simulink model "angleControllerValidation"  (R2021b)
settings: Solver=VariableStepAuto  StartTime=0.0  StopTime=10.0  RelTol=1e-3
values from neighbouring files (symbols this model uses):
  B_x = 12    [XthetaControllers.m]    (also in x_model_sheet.m)
  J_x = 0.13    [XthetaControllers.m]    (also in x_model_sheet.m)
  r_x = 75e-3    (= 0.075)    [XthetaControllers.m]    (also in x_model_sheet.m)
undefined symbols (not defined in the file or in its folder): cFrictionX, InitWireLength, InitXPos, k_ex, m_l, m_t, sFrictionX, Xref
settings Model: Creator=bosto  LastModifiedBy=bosto

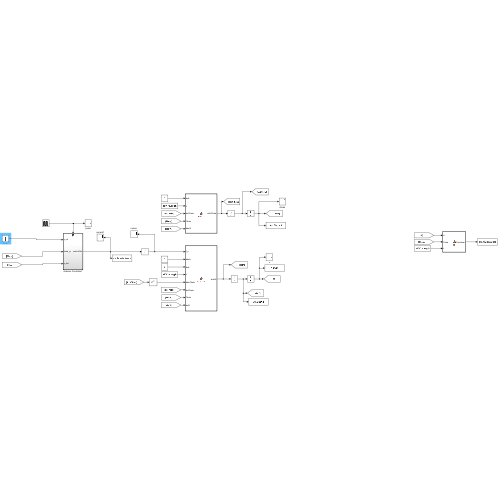
[thumbnail: Simulink's stored preview of the top-level diagram]
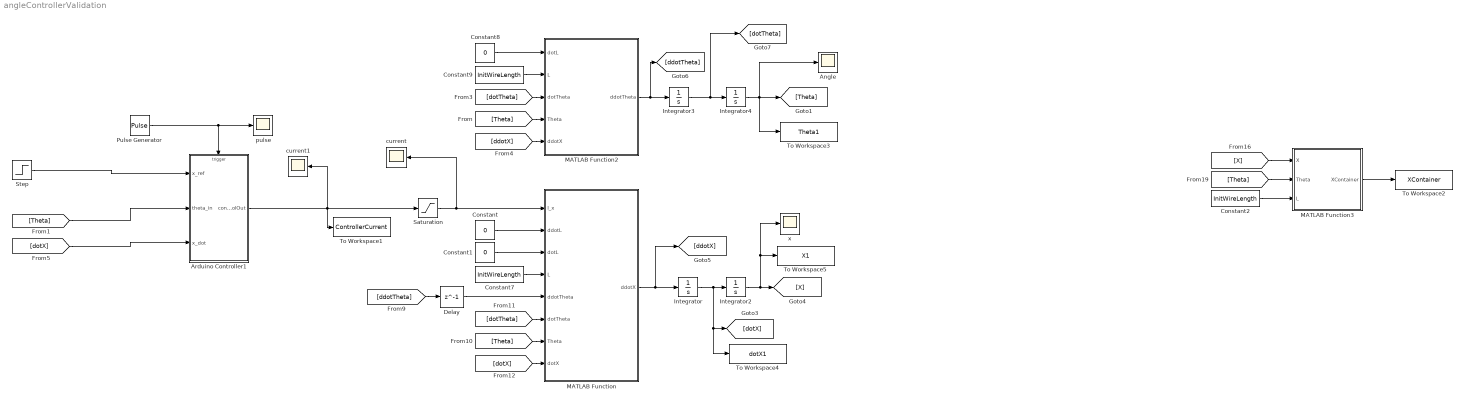
== system angleControllerValidation ==
  Angle : Scope
  Arduino Controller1 : Subsystem
  Constant : Constant  Value=0
  Constant1 : Constant  Value=0
  Constant2 : Constant  Value=InitWireLength
  Constant7 : Constant  Value=InitWireLength
  Constant8 : Constant  Value=0
  Constant9 : Constant  Value=InitWireLength
  Delay : Delay  DelayLength=1  InitialCondition=0
  Integrator : Integrator
  Integrator2 : Integrator  InitialCondition=InitXPos
  Integrator3 : Integrator
  Integrator4 : Integrator
  MATLAB Function : MATLAB Function  TreatAsAtomicUnit=on
  MATLAB Function2 : MATLAB Function  TreatAsAtomicUnit=on
  MATLAB Function3 : MATLAB Function  TreatAsAtomicUnit=on
  Pulse Generator : DiscretePulseGenerator  PulseType=Time based  Period=.012  PulseWidth=5
  Saturation : Saturate  UpperLimit=10  LowerLimit=-10
  Step : Step  Time=0  Before=InitXPos  After=Xref  SampleTime=0
  To Workspace1 : ToWorkspace  VariableName=ControllerCurrent  SampleTime=-1
  To Workspace2 : ToWorkspace  VariableName=XContainer  SampleTime=-1
  To Workspace3 : ToWorkspace  VariableName=Theta1  SampleTime=-1
  To Workspace4 : ToWorkspace  VariableName=dotX1  SampleTime=-1
  To Workspace5 : ToWorkspace  VariableName=X1  SampleTime=-1
  current : Scope
  current1 : Scope
  pulse : Scope
  x : Scope
  wires:
  [Theta] -> Arduino Controller1/2(theta_in)
  Integrator3/1 -> [dotTheta], Integrator4/1
  Constant7/1 -> MATLAB Function/4(L)
  Saturation/1 -> current/1, MATLAB Function/1(I_x)
  Arduino Controller1/1(controlOut) -> To Workspace1/1, current1/1, Saturation/1
  Step/1 -> Arduino Controller1/1(x_ref)
  [Theta] -> MATLAB Function3/2(Theta)
  Pulse Generator/1 -> pulse/1, Arduino Controller1/Trigger
  Constant2/1 -> MATLAB Function3/3(L)
  Delay/1 -> MATLAB Function/5(ddotTheta)
  MATLAB Function3/1(XContainer) -> To Workspace2/1
  [dotX] -> Arduino Controller1/3(x_dot)
  Constant8/1 -> MATLAB Function2/1(dotL)
  [ddotTheta] -> Delay/1
  Integrator/1 -> To Workspace4/1, [dotX], Integrator2/1
  Constant9/1 -> MATLAB Function2/2(L)
  Integrator4/1 -> Angle/1, To Workspace3/1, [Theta]
  [Theta] -> MATLAB Function2/4(Theta)
  MATLAB Function/1(ddotX) -> [ddotX], Integrator/1
  [ddotX] -> MATLAB Function2/5(ddotX)
  [dotX] -> MATLAB Function/8(dotX)
  Constant/1 -> MATLAB Function/2(ddotL)
  MATLAB Function2/1(ddotTheta) -> [ddotTheta], Integrator3/1
  Integrator2/1 -> x/1, To Workspace5/1, [X]
  [dotTheta] -> MATLAB Function/6(dotTheta)
  [dotTheta] -> MATLAB Function2/3(dotTheta)
  [X] -> MATLAB Function3/1(X)
  [Theta] -> MATLAB Function/7(Theta)
  Constant1/1 -> MATLAB Function/3(dotL)

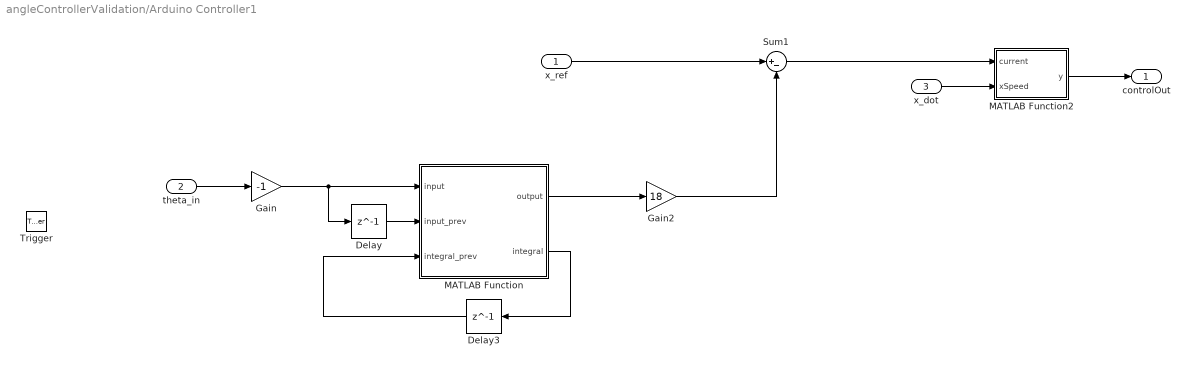
== system angleControllerValidation/Arduino Controller1 ==
  x_ref : Inport
  theta_in : Inport  Port=2
  x_dot : Inport  Port=3
  Trigger : TriggerPort  VariantControl=(inherit)  PortDimensions=1
  Delay : Delay  DelayLength=1  InitialCondition=0
  Delay3 : Delay  DelayLength=1  InitialCondition=0
  Gain : Gain  Gain=-1
  Gain2 : Gain  Gain=18
  MATLAB Function : MATLAB Function  TreatAsAtomicUnit=on
  MATLAB Function2 : MATLAB Function  TreatAsAtomicUnit=on
  Sum1 : Sum  Inputs=|+-
  controlOut : Outport
  wires:
  theta_in/1 -> Gain/1
  Delay/1 -> MATLAB Function/2(input_prev)
  MATLAB Function/2(integral) -> Delay3/1
  Delay3/1 -> MATLAB Function/3(integral_prev)
  MATLAB Function/1(output) -> Gain2/1
  Gain/1 -> Delay/1, MATLAB Function/1(input)
  MATLAB Function2/1(y) -> controlOut/1
  Sum1/1 -> MATLAB Function2/1(current)
  x_dot/1 -> MATLAB Function2/2(xSpeed)
  Gain2/1 -> Sum1/2
  x_ref/1 -> Sum1/1

== matlab function angleControllerValidation/MATLAB Function ==
  data: I_x input; ddotX output; ddotL input; dotL input; L input; ddotTheta input; dotTheta input; Theta input; dotX input; J_x parameter; r_x parameter double; k_ex parameter; m_t parameter; m_l parameter; B_x parameter; sFrictionX parameter; cFrictionX parameter
function ddotX = fcn5_10(I_x, ddotL, dotL, L, ddotTheta, dotTheta, Theta, dotX, J_x, r_x, k_ex, m_t, m_l, B_x,sFrictionX, cFrictionX)

if(norm(dotX)<0.05)
    friction = sFrictionX*sign(dotX);
else
    friction = B_x*dotX+cFrictionX*sign(dotX);
end



temp = I_x*k_ex/r_x;

temp = temp  - m_l*ddotL*sin(Theta);

temp= temp -2*m_l*dotL*dotTheta*cos(Theta);

temp = temp - m_l*L*ddotTheta*cos(Theta);

temp = temp + m_l*L*(dotTheta^2)*sin(Theta);

temp = temp - friction;

temp = temp/(m_t+m_l+J_x/(r_x^2));

ddotX = temp;

== matlab function angleControllerValidation/MATLAB Function2 ==
  data: ddotTheta output; dotL input; L input; dotTheta input; Theta input; ddotX input; g parameter
function ddotTheta = fcn5_7(dotL, L, dotTheta, Theta,ddotX,g)

temp = -2*dotL*dotTheta;

temp = temp - ddotX*cos(Theta);

temp = temp - g*sin(Theta);

temp = temp/L;

ddotTheta = temp;

== matlab function angleControllerValidation/MATLAB Function3 ==
  data: X input; XContainer output; Theta input; L input
function XContainer = fcn(X,Theta,L)

XContainer = X + sin(Theta)*L;

== matlab function angleControllerValidation/Arduino Controller1/MATLAB Function ==
  data: input input; output output; input_prev input; integral_prev input; integral output
function [output, integral]= parallelPID(input, input_prev, integral_prev)
P = .16;
I = 0;
D = 1;
deltaTime = .01;

proportional = input*P;
derivative = D*(input-input_prev)/deltaTime;
integral = integral_prev + I*input*deltaTime; 

output = proportional+derivative+integral;

end

== matlab function angleControllerValidation/Arduino Controller1/MATLAB Function2 ==
  data: current input; y output; xSpeed input
function y = fcn(current, xSpeed)
    if (abs(current) < 0.2)
        y = 0;
    elseif (xSpeed < 0)
        y = current - 2.21;
    
    elseif (xSpeed > 0)
        y = current + 2.21;
    else 
        y = current;
    end
end
